simulink model "zadanie_dodatkowe_sim"  (R2022b)
settings: Solver=VariableStepAuto  StartTime=0.0  StopTime=10  RelTol=1e-3
values from neighbouring files (symbols this model uses):
  k1 = K(1)    [zad3.m]    (also in zadanie_dodatkowe.m)
  k2 = K(2)    [zad3.m]    (also in zadanie_dodatkowe.m)
  k3 = K(3)    [zad3.m]    (also in zadanie_dodatkowe.m)
  k4 = K(4)    [zadanie_dodatkowe.m]
settings Model: Creator=Mat  LastModifiedBy=Mat

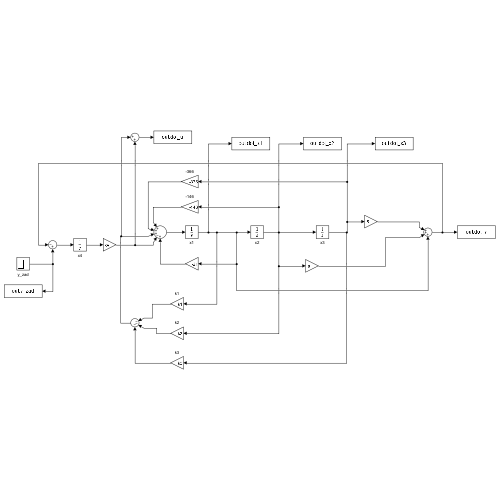
[thumbnail: Simulink's stored preview of the top-level diagram]
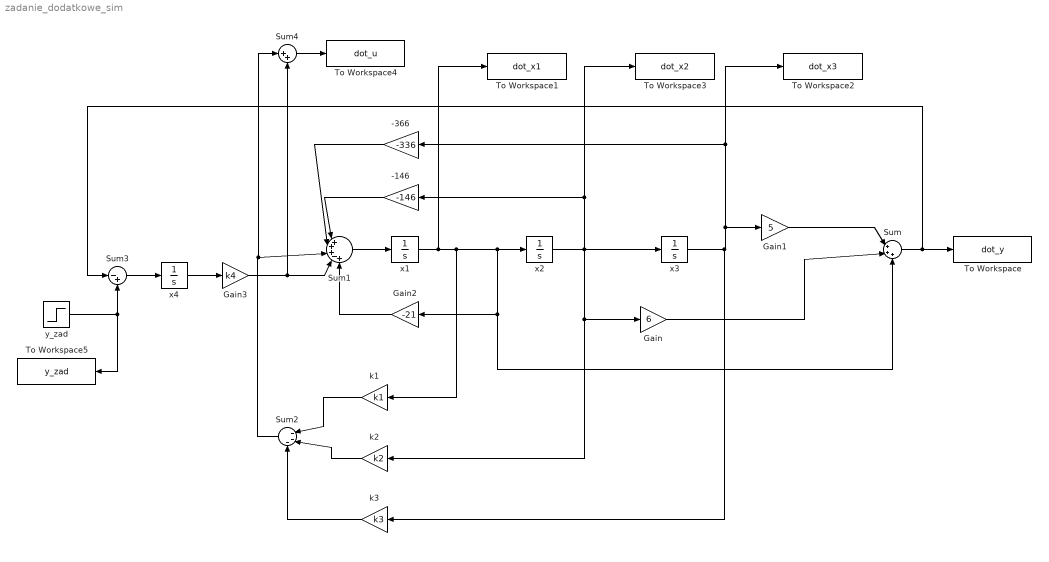
== system zadanie_dodatkowe_sim ==
  -146 : Gain  Gain=-146
  -366 : Gain  Gain=-336
  Gain : Gain  Gain=6
  Gain1 : Gain  Gain=5
  Gain2 : Gain  Gain=-21
  Gain3 : Gain  Gain=k4
  Sum : Sum  Inputs=|+++
  Sum1 : Sum  Inputs=|+++-+
  Sum2 : Sum  Inputs=|---
  Sum3 : Sum  Inputs=|-+
  Sum4 : Sum  Inputs=|++
  To Workspace : ToWorkspace  VariableName=dot_y  SaveFormat=Timeseries  SampleTime=-1
  To Workspace1 : ToWorkspace  VariableName=dot_x1  SaveFormat=Timeseries  SampleTime=-1
  To Workspace2 : ToWorkspace  VariableName=dot_x3  SaveFormat=Timeseries  SampleTime=-1
  To Workspace3 : ToWorkspace  VariableName=dot_x2  SaveFormat=Timeseries  SampleTime=-1
  To Workspace4 : ToWorkspace  VariableName=dot_u  SaveFormat=Timeseries  SampleTime=-1
  To Workspace5 : ToWorkspace  VariableName=y_zad  SaveFormat=Timeseries  SampleTime=-1
  k1 : Gain  Gain=k1
  k2 : Gain  Gain=k2
  k3 : Gain  Gain=k3
  x{1..4} (4 alike) : Integrator
  y_zad : Step  SampleTime=0
  wires:
  -366/1 -> Sum1/2
  Gain/1 -> Sum/2
  x3/1 -> k3/1, Gain1/1, To Workspace2/1, -366/1
  x1/1 -> k1/1, Gain2/1, Sum/3, x2/1, To Workspace1/1
  k1/1 -> Sum2/1
  Sum2/1 -> Sum4/1, Sum1/3
  k3/1 -> Sum2/3
  k2/1 -> Sum2/2
  Sum1/1 -> x1/1
  Sum/1 -> To Workspace/1, Sum3/1
  -146/1 -> Sum1/1
  Gain1/1 -> Sum/1
  x2/1 -> To Workspace3/1, -146/1, x3/1, Gain/1, k2/1
  Gain2/1 -> Sum1/5
  Sum3/1 -> x4/1
  Gain3/1 -> Sum4/2, Sum1/4
  x4/1 -> Gain3/1
  y_zad/1 -> To Workspace5/1, Sum3/2
  Sum4/1 -> To Workspace4/1
